simulink model "Sim7"  (R2021b)
settings: Solver=FixedStepDiscrete  StartTime=0.0  StopTime=1  FixedStep=1e-6  RelTol=1e-3  EnableMultiTasking=on
InitFcn:
  | clc
  | Ts=1e-6;
  | ts=Ts;
  | Td=Ts;
  | disp(sprintf('Ts = %f',Ts))
  |  %1/fs = sampling period;
  | Ts = Td;
  | Tch = Td;
  | 
  | %harmonics
  | kh=0;
  | 
  | % PLL
  | Tset = 0.1; % settling time
  | zeta = 0.707;   % damping ratio (optimized for best response of the second order TF
  | 
  | %grid params
  | tha = 0;
  | kh = 0;
  | V1 = 230;
  | fg = 50;
  | 
  | %freq var
  | onoff = 0;
  | onoff_faults = 1;
  | fperiod = 2;
  | fmin = 48;
  | fmax = 52;
undefined symbols (not defined in the file or in its folder): DiscIntNeverNeededParam
libraries: spsThreePhaseSeriesRLCBranchLib x8, powerlib_extras x5, spsThreePhaseVIMeasurementLib x5, spsSeriesRLCBranchLib x3, spsUniversalBridgeLib x3, spsGroundLib x2, spsDCVoltageSourceLib x2, spsThreePhaseBreakerLib x2, spspowerguiLib x1
(part 1 of 2)
settings Model: SimulationMode=accelerator  Creator=juancho  LastModifiedBy=sebastian
settings SolverCC: AlgebraicLoopSolver=TrustRegion
settings DataIOCC: SaveFormat=Array  SignalLoggingSaveFormat=ModelDataLogs  SaveOutput=off  SignalLogging=off  SaveTime=off  ReturnWorkspaceOutputs=off
settings OptimizationCC: ExpressionDepthLimit=2147483647  LifeSpan=inf
settings DebuggingCC: UnderspecifiedInitializationDetection=Classic  MergeDetectMultiDrivingBlocksExec=none  SolverPrmCheckMsg=warning  InheritedTsInSrcMsg=error  FcnCallInpInsideContextMsg=warning  AllowSymbolicDim=off  StateNameClashWarn=warning  SFUnexpectedBacktrackingDiag=warning  SFNoUnconditionalDefaultTransitionDiag=warning  SFExecutionAtInitializationDiag=none  SFMachineParentedDataDiag=warning  ArithmeticOperatorsInVariantConditions=warning
settings HardwareCC: ProdBitPerPointer=32  ProdBitPerSizeT=32  ProdBitPerPtrDiffT=32  ProdLargestAtomicFloat=None  ProdIntDivRoundTo=Undefined  ProdEndianess=Unspecified  ProdWordSize=32  ProdHWDeviceType=32-bit Generic
settings ModelReferenceCC: PropagateSignalLabelsOutOfModel=off
settings SFSimCC: SimUseLocalCustomCode=off  CustomCodeUndefinedFunction=UseInterfaceOnly
settings RTWCC: RTWUseLocalCustomCode=off
settings CodeAppCC: StateflowObjectComments=on
settings GRTTargetCC: TargetLangStandard=C89/C90 (ANSI)  CombineOutputUpdateFcns=off  GRTInterface=on
settings ConfigComp: CovMetricSettings=dw  CovSaveCumulativeToWorkspaceVar=on  CovSaveSingleToWorkspaceVar=on  CovExternalEMLEnable=off  CovSFcnEnable=off
settings SimscapeCC: SimscapeNormalizeSystem=off

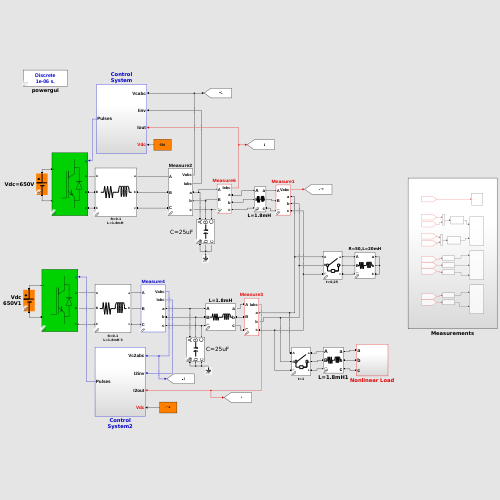
[thumbnail: Simulink's stored preview of the top-level diagram]
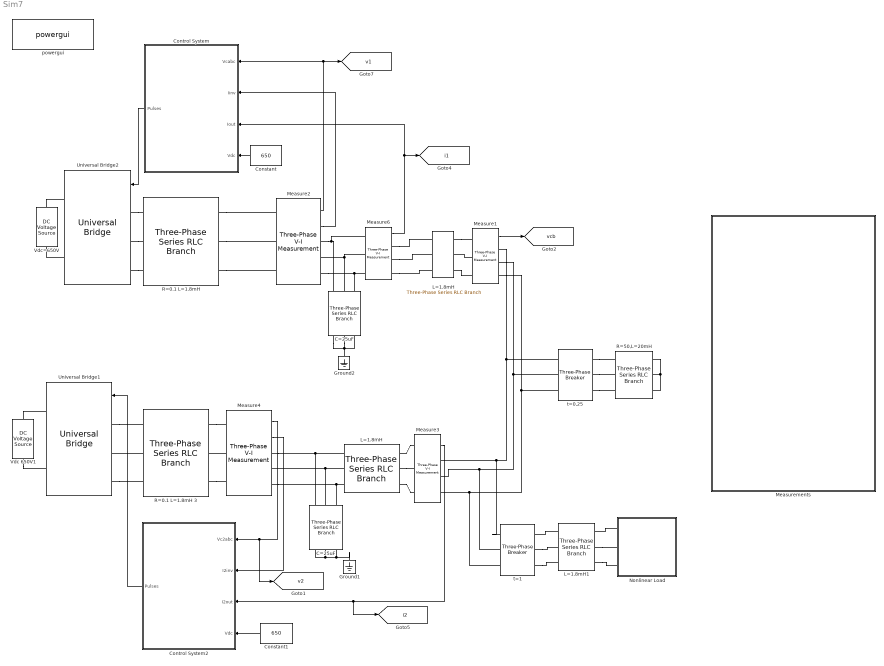
== system Sim7 ==
  C=25uF : spsThreePhaseSeriesRLCBranchLib/Three-Phase Series RLC Branch  LConnTagsString=A|B|C  RConnTagsString=A|B|C  BranchType=C  Resistance=1.0  Inductance=1e-3  Capacitance=25e-6  Measurements=None
  "C=25uF " : spsThreePhaseSeriesRLCBranchLib/Three-Phase Series RLC Branch  LConnTagsString=A|B|C  RConnTagsString=A|B|C  BranchType=C  Resistance=1.0  Inductance=1e-3  Capacitance=25e-6  Measurements=None
  Constant : Constant  Value=650
  Constant1 : Constant  Value=650
  Control System : Subsystem
  Control System2 : Subsystem
  Ground1 : spsGroundLib/Ground  LConnTagsString=a
  Ground2 : spsGroundLib/Ground  LConnTagsString=a
  L=1.8mH : spsThreePhaseSeriesRLCBranchLib/Three-Phase Series RLC Branch  LConnTagsString=A|B|C  RConnTagsString=A|B|C  BranchType=RL  Resistance=0.1  Inductance=1.8e-3  Capacitance=1.0  Measurements=None
  "L=1.8mH " : spsThreePhaseSeriesRLCBranchLib/Three-Phase Series RLC Branch  LConnTagsString=A|B|C  RConnTagsString=A|B|C  BranchType=RL  Resistance=0.1  Inductance=1.8e-3  Capacitance=1.0  Measurements=None
  L=1.8mH1 : spsThreePhaseSeriesRLCBranchLib/Three-Phase Series RLC Branch  LConnTagsString=A|B|C  RConnTagsString=A|B|C  BranchType=RL  Resistance=0.1  Inductance=(1.8e-3)  Capacitance=1.0  Measurements=None
  Measure1 : spsThreePhaseVIMeasurementLib/Three-Phase V-I Measurement  VoltageMeasurement=phase-to-ground  SetLabelV=off  LabelV=V1  Vpu=off  VpuLL=off  CurrentMeasurement=no  SetLabelI=off  LabelI=I1  Ipu=off  Pbase=1e3  Vbase=380  OutputType=Magnitude  PhasorSimulation=off  PSBequivalent=0
  Measure2 : spsThreePhaseVIMeasurementLib/Three-Phase V-I Measurement  VoltageMeasurement=phase-to-ground  SetLabelV=off  LabelV=V1  Vpu=off  VpuLL=off  CurrentMeasurement=yes  SetLabelI=off  LabelI=I1  Ipu=off  Pbase=1e3  Vbase=380  OutputType=Magnitude  PhasorSimulation=off  PSBequivalent=0
  Measure3 : spsThreePhaseVIMeasurementLib/Three-Phase V-I Measurement  VoltageMeasurement=no  SetLabelV=off  LabelV=V1  Vpu=off  VpuLL=off  CurrentMeasurement=yes  SetLabelI=off  LabelI=I1  Ipu=off  Pbase=1e3  Vbase=380  OutputType=Magnitude  PhasorSimulation=off  PSBequivalent=0
  Measure4 : spsThreePhaseVIMeasurementLib/Three-Phase V-I Measurement  VoltageMeasurement=phase-to-ground  SetLabelV=off  LabelV=V1  Vpu=off  VpuLL=off  CurrentMeasurement=yes  SetLabelI=off  LabelI=I1  Ipu=off  Pbase=1e3  Vbase=380  OutputType=Magnitude  PhasorSimulation=off  PSBequivalent=0
  Measure6 : spsThreePhaseVIMeasurementLib/Three-Phase V-I Measurement  VoltageMeasurement=no  SetLabelV=off  LabelV=V1  Vpu=off  VpuLL=off  CurrentMeasurement=yes  SetLabelI=off  LabelI=I1  Ipu=off  Pbase=1e3  Vbase=380  OutputType=Magnitude  PhasorSimulation=off  PSBequivalent=0
  Measurements : Subsystem
  Nonlinear Load : Subsystem
  "R=0.1 L=1.8mH " : spsThreePhaseSeriesRLCBranchLib/Three-Phase Series RLC Branch  LConnTagsString=A|B|C  RConnTagsString=A|B|C  BranchType=RL  Resistance=0.1  Inductance=1.8e-3  Capacitance=1.0  Measurements=None
  R=0.1 L=1.8mH 3 : spsThreePhaseSeriesRLCBranchLib/Three-Phase Series RLC Branch  LConnTagsString=A|B|C  RConnTagsString=A|B|C  BranchType=RL  Resistance=0.1  Inductance=1.8e-3  Capacitance=1.0  Measurements=None
  R=50,L=20mH : spsThreePhaseSeriesRLCBranchLib/Three-Phase Series RLC Branch  LConnTagsString=A|B|C  RConnTagsString=A|B|C  BranchType=RL  Resistance=50  Inductance=20e-3  Capacitance=1.0  Measurements=None
  Universal Bridge1 : spsUniversalBridgeLib/Universal Bridge  Arms=3  SnubberResistance=1e5  SnubberCapacitance=inf  Device=IGBT / Diodes  Ron=1e-3  Lon=0  ForwardVoltages="[  0  0  ]"  ForwardVoltage=0  GTOparameters=[ 10e-6 , 20e-6 ]  IGBTparameters=[ 1e-6 , 2e-6]  Measurements=None  Measurements_2=None  converterType=Rectifier
  Universal Bridge2 : spsUniversalBridgeLib/Universal Bridge  Arms=3  SnubberResistance=1e5  SnubberCapacitance=inf  Device=IGBT / Diodes  Ron=1e-3  Lon=0  ForwardVoltages="[  0  0  ]"  ForwardVoltage=0  GTOparameters=[ 10e-6 , 20e-6 ]  IGBTparameters=[ 1e-6 , 2e-6 ]  Measurements=None  Measurements_2=None  converterType=Rectifier
  Vdc 650V1 : spsDCVoltageSourceLib/DC Voltage Source  Description=source block  Amplitude=650  Measurements=None
      settings: AttributesFormatString=\n
  Vdc=650V : spsDCVoltageSourceLib/DC Voltage Source  Description=source block  Amplitude=650  Measurements=None
      settings: AttributesFormatString=\n
  powergui : spspowerguiLib/powergui  Priority=1  SimulationMode=Discrete  SampleTime=1e-6  frequency=60  Iterations=50  frequencyindice=0  Pbase=100e6  ErrMax=1e-4  UnitsV=kV  UnitsW=MW  buscounter=0  FunctionMessages=off  echomessages=off  EnableUseOfTLC=off  CurrentSourceSwitches=off  DisableSnubberDevices=off  DisableRonSwitches=off  DisableVfSwitches=off  DisplayEquations=off  AutomaticDiscreteSolvers=off  SolverType=Tustin  Interpol=off  ExternalGateDelay=off  methode=off  Ts=0  x0status=blocks  SPID=off  SwTol=0  HookPort=off  NonlinearTolerance=1e-4  nMaxIteration=100  ContinueOnMaxIteration=off  RestoreLinks=warning  ResistiveCurrentMeasurement=off  Frange=[0:2:500]  Ylog=off  Xlog=on  ShowGrid=off  save=off  variable=ZData  structure=vload  ZoomFFT=off  StartTime=4.8  cycles=9  DisplayStyle=1  fundamental=49.953  FreqAxis=on  MaxFrequency=1000  frequencyindicesteady=1  RmsSteady=1  display=off
  "t=0,25 " : spsThreePhaseBreakerLib/Three-Phase Breaker  InitialState=open  SwitchA=on  SwitchB=on  SwitchC=on  SwitchTimes=0.25  External=off  BreakerResistance=0.001  SnubberResistance=1e6  SnubberCapacitance=inf  Measurements=None
  t=1 : spsThreePhaseBreakerLib/Three-Phase Breaker  InitialState=open  SwitchA=on  SwitchB=on  SwitchC=on  SwitchTimes=1  External=off  BreakerResistance=0.001  SnubberResistance=1e6  SnubberCapacitance=inf  Measurements=Breaker voltages and currents
  tag scope: i1=global, i2=global, v1=global, v2=global, vcb=global
  wires:
  Control System/1(Pulses) -> Universal Bridge2/1
  Constant/1 -> Control System/4(Vdc)
  Measure2/1 -> Control System/1(Vcabc), [v1]
  Measure4/1 -> [v2], Control System2/1(Vc2abc)
  Control System2/1(Pulses) -> Universal Bridge1/1
  Measure4/2 -> Control System2/2(I2inv)
  Measure3/1 -> [i2], Control System2/3(I2out)
  Constant1/1 -> Control System2/4(Vdc)
  Measure2/2 -> Control System/2(Iinv)
  Measure6/1 -> [i1], Control System/3(Iout)
  Measure1/1 -> [vcb]
  connections:
  Universal Bridge2/LConn3 -- "R=0.1 L=1.8mH "/LConn3
  Universal Bridge2/LConn1 -- "R=0.1 L=1.8mH "/LConn1
  Universal Bridge2/LConn2 -- "R=0.1 L=1.8mH "/LConn2
  Universal Bridge2/RConn2 -- Vdc=650V/LConn1
  Vdc=650V/RConn1 -- Universal Bridge2/RConn1
  "R=0.1 L=1.8mH "/RConn1 -- Measure2/LConn1
  "R=0.1 L=1.8mH "/RConn2 -- Measure2/LConn2
  "R=0.1 L=1.8mH "/RConn3 -- Measure2/LConn3
  "C=25uF "/RConn2 -- Ground2/LConn1 -- "C=25uF "/RConn1 -- "C=25uF "/RConn3
  Measure1/RConn2 -- t=1/LConn2 -- Measure3/RConn2 -- "t=0,25 "/LConn2
  Measure1/RConn3 -- t=1/LConn3 -- Measure3/RConn3 -- "t=0,25 "/LConn3
  Universal Bridge1/LConn1 -- R=0.1 L=1.8mH 3/LConn1
  R=0.1 L=1.8mH 3/LConn2 -- Universal Bridge1/LConn2
  Universal Bridge1/LConn3 -- R=0.1 L=1.8mH 3/LConn3
  R=0.1 L=1.8mH 3/RConn1 -- Measure4/LConn1
  Measure4/LConn2 -- R=0.1 L=1.8mH 3/RConn2
  R=0.1 L=1.8mH 3/RConn3 -- Measure4/LConn3
  Measure4/RConn1 -- L=1.8mH/LConn1 -- C=25uF/LConn1
  L=1.8mH/LConn2 -- Measure4/RConn2 -- C=25uF/LConn2
  L=1.8mH/RConn1 -- Measure3/LConn1
  L=1.8mH/RConn2 -- Measure3/LConn2
  L=1.8mH/RConn3 -- Measure3/LConn3
  Measure1/RConn1 -- "t=0,25 "/LConn1 -- t=1/LConn1 -- Measure3/RConn1
  Measure2/RConn3 -- Measure6/LConn3 -- "C=25uF "/LConn3
  Measure2/RConn1 -- Measure6/LConn1 -- "C=25uF "/LConn1
  "C=25uF "/LConn2 -- Measure6/LConn2 -- Measure2/RConn2
  C=25uF/RConn3 -- C=25uF/RConn1 -- C=25uF/RConn2 -- Ground1/LConn1
  Measure4/RConn3 -- L=1.8mH/LConn3 -- C=25uF/LConn3
  Vdc 650V1/LConn1 -- Universal Bridge1/RConn2
  Vdc 650V1/RConn1 -- Universal Bridge1/RConn1
  R=50,L=20mH/RConn2 -- R=50,L=20mH/RConn1 -- R=50,L=20mH/RConn3
  "t=0,25 "/RConn1 -- R=50,L=20mH/LConn1
  "t=0,25 "/RConn2 -- R=50,L=20mH/LConn2
  "L=1.8mH "/RConn1 -- Measure1/LConn1
  Measure1/LConn2 -- "L=1.8mH "/RConn2
  "L=1.8mH "/RConn3 -- Measure1/LConn3
  Measure6/RConn1 -- "L=1.8mH "/LConn1
  Measure6/RConn2 -- "L=1.8mH "/LConn2
  Measure6/RConn3 -- "L=1.8mH "/LConn3
  "t=0,25 "/RConn3 -- R=50,L=20mH/LConn3
  L=1.8mH1/RConn2 -- Nonlinear Load/LConn2
  L=1.8mH1/LConn1 -- t=1/RConn1
  t=1/RConn2 -- L=1.8mH1/LConn2
  Nonlinear Load/LConn1 -- L=1.8mH1/RConn1
  L=1.8mH1/RConn3 -- Nonlinear Load/LConn3
  t=1/RConn3 -- L=1.8mH1/LConn3

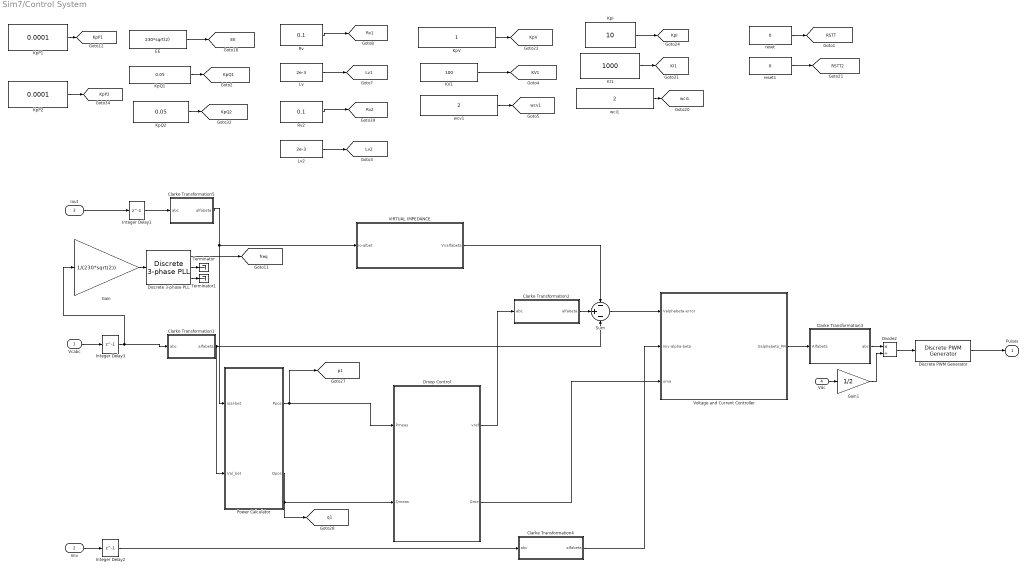
== system Sim7/Control System ==
  Vcabc : Inport
  Iinv : Inport  Port=2
  Iout : Inport  Port=3
  Vdc : Inport  Port=4
  Clarke Transformation3 : Subsystem
  Clarke Transformation1 : Subsystem
  Clarke Transformation2 : Subsystem
  Clarke Transformation4 : Subsystem
  Clarke Transformation5 : Subsystem
  Discrete 3-phase PLL : powerlib_extras/Discrete  Control Blocks/Discrete 3-phase PLL  Fmin=45  Par_Init=[0 50]  ParK=[ 180 3200 1 ]  Ts=1e-6  AGC=off
      settings: SourceProductBaseCode=PS
  Discrete PWM Generator : powerlib_extras/Discrete  Control Blocks/Discrete PWM Generator  GeneratorMode="3-arm  bridge (6 pulses)"  Fc=1e4  Ts=1e-6  Internal=off  mIndex=0.4  Freq=60  Phase=0
      settings: SourceProductBaseCode=PS
  Divide2 : Product  Inputs=*/  SampleTime=Ts
  Droop Control : Subsystem
  EE : Constant  Value=230*sqrt(2)
  Gain : Gain  Gain=1/(230*sqrt(2))
  Gain1 : Gain  Gain=1/2  SampleTime=Ts
  Integer Delay1 : Delay  DelayLength=1  SampleTime=1e-6
  Integer Delay2 : Delay  DelayLength=1  SampleTime=1e-6
  Integer Delay3 : Delay  DelayLength=1  SampleTime=1e-6
  KI1 : Constant  Value=1000
  KV1 : Constant  Value=100
  KpI : Constant  Value=10
  KpP1 : Constant  Value=0.0001
  KpP2 : Constant  Value=0.0001
  KpQ1 : Constant  Value=0.05  VectorParams1D=off
  KpQ2 : Constant  Value=0.05  VectorParams1D=off
  KpV : Constant
  Lv : Constant  Value=2e-3
  Lv2 : Constant  Value=2e-3
  Power Calculator : Subsystem
  Rv : Constant  Value=0.1
  Rv2 : Constant  Value=0.1
  Sum : Sum  Inputs=-+-  SampleTime=Ts
  Terminator : Terminator
  Terminator1 : Terminator
  VIRTUAL IMPEDANCE : Subsystem
  "Voltage and Current Controller " : Subsystem
  reset : Constant  Value=0
  reset1 : Constant  Value=0
  wci1 : Constant  Value=2
  wcv1 : Constant  Value=2
  Pulses : Outport  SampleTime=1e-6
  tag scope: EE=global, KI1=global, KV1=global, KpI=global, KpP1=global, KpP2=global, KpQ1=global, KpQ2=global, KpV=global, Lv1=global, Lv2=global, RSTT2=global, RSTT=global, Rv1=global, Rv2=global, freq=global, p1=global, q1=global, wci1=global, wcv1=global
  wires:
  Lv/1 -> [Lv1]
  Rv/1 -> [Rv1]
  KpP1/1 -> [KpP1]
  KpQ1/1 -> [KpQ1]
  EE/1 -> [EE]
  reset/1 -> [RSTT]
  Iinv/1 -> Integer Delay2/1
  Iout/1 -> Integer Delay1/1
  Vcabc/1 -> Integer Delay3/1
  Vdc/1 -> Gain1/1
  VIRTUAL IMPEDANCE/1(Vvalfabeta) -> Sum/1
  Clarke Transformation2/1(alfabeta) -> Sum/2
  Clarke Transformation5/1(alfabeta) -> Power Calculator/1(ioal-bet), VIRTUAL IMPEDANCE/1(io-albet)
  Clarke Transformation1/1(alfabeta) -> Sum/3, Power Calculator/2(Val_bet)
  Droop Control/2(Ome) -> "Voltage and Current Controller "/3(ome)
  Divide2/1 -> Discrete PWM Generator/1
  Gain1/1 -> Divide2/2
  Clarke Transformation3/1(abc) -> Divide2/1
  Discrete PWM Generator/1 -> Pulses/1
  Integer Delay2/1 -> Clarke Transformation4/1(abc)
  Integer Delay3/1 -> Clarke Transformation1/1(abc), Gain/1
  Integer Delay1/1 -> Clarke Transformation5/1(abc)
  Droop Control/1(vref) -> Clarke Transformation2/1(abc)
  Power Calculator/1(Ppos) -> [p1], Droop Control/1(Pmeas)
  Power Calculator/2(Qpos) -> Droop Control/2(Qmeas), [q1]
  reset1/1 -> [RSTT2]
  "Voltage and Current Controller "/1(Ualphabeta_PR) -> Clarke Transformation3/1(Alfabeta)
  Clarke Transformation4/1(alfabeta) -> "Voltage and Current Controller "/2(Iinv-alpha-beta)
  Sum/1 -> "Voltage and Current Controller "/1(Valphabeta-error)
  KpV/1 -> [KpV]
  KpI/1 -> [KpI]
  KI1/1 -> [KI1]
  KV1/1 -> [KV1]
  wcv1/1 -> [wcv1]
  wci1/1 -> [wci1]
  Gain/1 -> Discrete 3-phase PLL/1
  Discrete 3-phase PLL/1 -> [freq]
  KpQ2/1 -> [KpQ2]
  KpP2/1 -> [KpP2]
  Lv2/1 -> [Lv2]
  Rv2/1 -> [Rv2]
  Discrete 3-phase PLL/2 -> Terminator/1
  Discrete 3-phase PLL/3 -> Terminator1/1

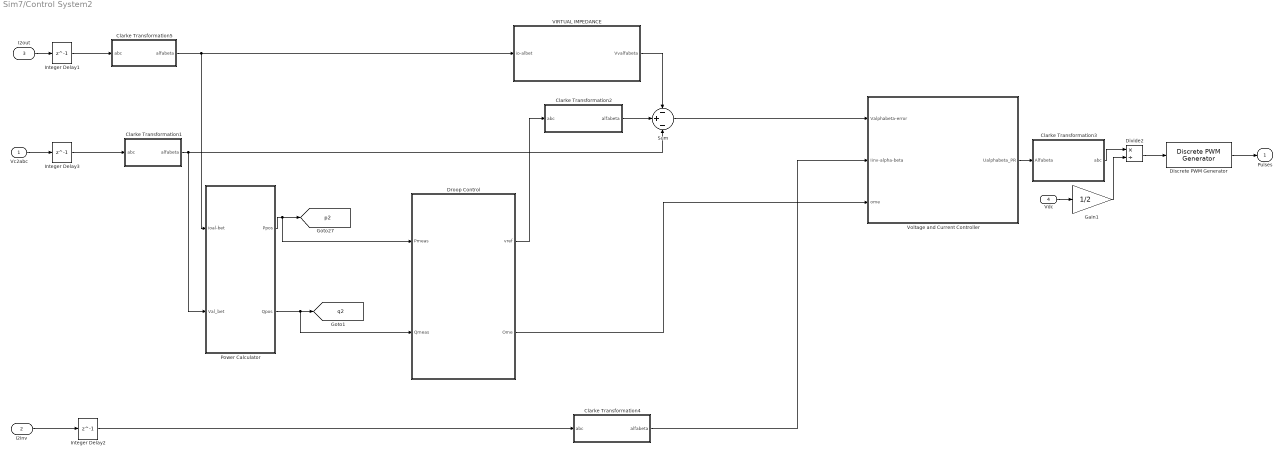
== system Sim7/Control System2 ==
  Vc2abc : Inport
  I2inv : Inport  Port=2
  I2out : Inport  Port=3
  Vdc : Inport  Port=4
  Clarke Transformation3 : Subsystem
  Clarke Transformation1 : Subsystem
  Clarke Transformation2 : Subsystem
  Clarke Transformation4 : Subsystem
  Clarke Transformation5 : Subsystem
  Discrete PWM Generator : powerlib_extras/Discrete  Control Blocks/Discrete PWM Generator  GeneratorMode="3-arm  bridge (6 pulses)"  Fc=1e4  Ts=1e-6  Internal=off  mIndex=0.4  Freq=60  Phase=0
      settings: SourceProductBaseCode=PS
  Divide2 : Product  Inputs=*/  SampleTime=Ts
  Droop Control : Subsystem
  Gain1 : Gain  Gain=1/2  SampleTime=Ts
  Integer Delay1 : Delay  DelayLength=1  SampleTime=1e-6
  Integer Delay2 : Delay  DelayLength=1  SampleTime=1e-6
  Integer Delay3 : Delay  DelayLength=1  SampleTime=1e-6
  Power Calculator : Subsystem
  Sum : Sum  Inputs=-+-  SampleTime=Ts
  VIRTUAL IMPEDANCE : Subsystem
  Voltage and Current Controller : Subsystem
  Pulses : Outport  SampleTime=1e-6
  tag scope: p2=global, q2=global
  wires:
  Droop Control/2(Ome) -> Voltage and Current Controller/3(ome)
  Clarke Transformation1/1(alfabeta) -> Sum/3, Power Calculator/2(Val_bet)
  Clarke Transformation3/1(abc) -> Divide2/1
  Clarke Transformation2/1(alfabeta) -> Sum/2
  VIRTUAL IMPEDANCE/1(Vvalfabeta) -> Sum/1
  Gain1/1 -> Divide2/2
  Vc2abc/1 -> Integer Delay3/1
  I2out/1 -> Integer Delay1/1
  Integer Delay2/1 -> Clarke Transformation4/1(abc)
  I2inv/1 -> Integer Delay2/1
  Vdc/1 -> Gain1/1
  Divide2/1 -> Discrete PWM Generator/1
  Discrete PWM Generator/1 -> Pulses/1
  Integer Delay3/1 -> Clarke Transformation1/1(abc)
  Integer Delay1/1 -> Clarke Transformation5/1(abc)
  Clarke Transformation5/1(alfabeta) -> VIRTUAL IMPEDANCE/1(io-albet), Power Calculator/1(ioal-bet)
  Power Calculator/1(Ppos) -> Droop Control/1(Pmeas), [p2]
  Power Calculator/2(Qpos) -> Droop Control/2(Qmeas), [q2]
  Droop Control/1(vref) -> Clarke Transformation2/1(abc)
  Voltage and Current Controller/1(Ualphabeta_PR) -> Clarke Transformation3/1(Alfabeta)
  Clarke Transformation4/1(alfabeta) -> Voltage and Current Controller/2(Iinv-alpha-beta)
  Sum/1 -> Voltage and Current Controller/1(Valphabeta-error)

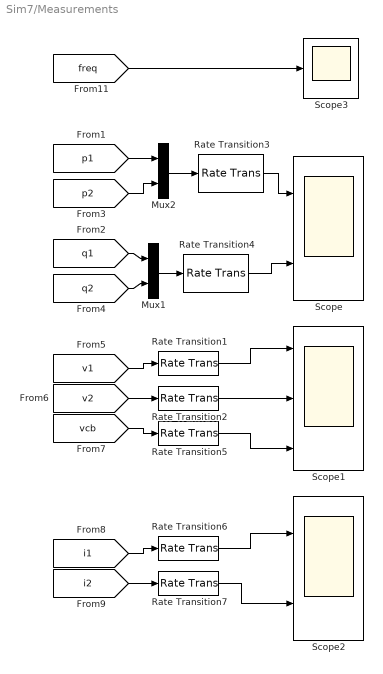
== system Sim7/Measurements ==
  Mux1 : Mux  Inputs=2
  Mux2 : Mux  Inputs=2
  Rate Transition{1..7} (7 alike) : RateTransition  OutPortSampleTime=1e-4
  Scope : Scope  NumInputPorts=2
  Scope1 : Scope  NumInputPorts=3
  Scope2 : Scope  NumInputPorts=2
  Scope3 : Scope
  wires:
  [p2] -> Mux2/2
  Rate Transition2/1 -> Scope1/2
  Rate Transition7/1 -> Scope2/2
  [v1] -> Rate Transition1/1
  Rate Transition1/1 -> Scope1/1
  [v2] -> Rate Transition2/1
  Rate Transition5/1 -> Scope1/3
  [q1] -> Mux1/1
  [p1] -> Mux2/1
  [i1] -> Rate Transition6/1
  Rate Transition3/1 -> Scope/1
  Mux1/1 -> Rate Transition4/1
  [q2] -> Mux1/2
  Mux2/1 -> Rate Transition3/1
  Rate Transition4/1 -> Scope/2
  Rate Transition6/1 -> Scope2/1
  [i2] -> Rate Transition7/1
  [vcb] -> Rate Transition5/1
  [freq] -> Scope3/1

== system Sim7/Nonlinear Load ==
  84uH : spsSeriesRLCBranchLib/Series RLC Branch  LConnTagsString=__new0  RConnTagsString=__new0  BranchType=L  Resistance=1  Inductance=84e-6  SetiL0=off  InitialCurrent=0  Capacitance=1e-6  Setx0=off  InitialVoltage=0  Measurements=None
  C 235uF : spsSeriesRLCBranchLib/Series RLC Branch  LConnTagsString=__new0  RConnTagsString=__new0  BranchType=C  Resistance=10e3  Inductance=[]  SetiL0=off  InitialCurrent=0  Capacitance=235e-6  Setx0=off  InitialVoltage=0  Measurements=None
  R 50 Ohms : spsSeriesRLCBranchLib/Series RLC Branch  LConnTagsString=__new0  RConnTagsString=__new0  BranchType=R  Resistance=50  Inductance=1.8e-3  SetiL0=off  InitialCurrent=0  Capacitance=[]  Setx0=off  InitialVoltage=0  Measurements=None
  Universal Bridge : spsUniversalBridgeLib/Universal Bridge  Arms=3  SnubberResistance=1e5  SnubberCapacitance=1e-6  Device=Diodes  Ron=1e-3  Lon=0  ForwardVoltages="[  0  0  ]"  ForwardVoltage=0.8  GTOparameters=[ 10e-6 , 20e-6 ]  IGBTparameters=[ 1e-6 , 2e-6 ]  Measurements=All voltages and currents  Measurements_2=None  converterType=Rectifier
  a : PMIOPort  Side=Left
  b : PMIOPort  Port=2  Side=Left
  c : PMIOPort  Port=3  Side=Left
  connections:
  C 235uF/LConn1 -- R 50 Ohms/RConn1 -- Universal Bridge/RConn2
  R 50 Ohms/LConn1 -- 84uH/LConn1 -- C 235uF/RConn1
  Universal Bridge/LConn1 -- a/RConn1
  Universal Bridge/LConn3 -- c/RConn1
  Universal Bridge/LConn2 -- b/RConn1
  84uH/RConn1 -- Universal Bridge/RConn1

== system Sim7/Control System/Clarke Transformation3 ==
  Alfabeta : Inport  SampleTime=Ts
  A : Fcn  Expr=sqrt(2/3)*u[1]  SampleTime=Ts
  B : Fcn  Expr=sqrt(2/3)*((-1/2)*u[1] + (sqrt(3)/2)*u[2])  SampleTime=Ts
  C : Fcn  Expr=sqrt(2/3)*((-1/2)*u[1] - (sqrt(3)/2)*u[2])  SampleTime=Ts
  Mux1 : Mux  Inputs=3
  abc : Outport  SampleTime=Ts
  wires:
  C/1 -> Mux1/3
  Alfabeta/1 -> C/1, B/1, A/1
  B/1 -> Mux1/2
  A/1 -> Mux1/1
  Mux1/1 -> abc/1

== system Sim7/Control System/Clarke Transformation1 ==
  abc : Inport  SampleTime=Ts
  Clarke to Beta : Fcn  Expr=sqrt(2/3)*(0*u[1]+(sqrt(3)/2)*u[2]-(sqrt(3)/2)*u[3])  SampleTime=Ts
  Clarke to alpha : Fcn  Expr=sqrt(2/3)*(u[1]-(1/2)*u[2]-(1/2)*u[3])  SampleTime=Ts
  Mux1 : Mux  Inputs=2
  alfabeta : Outport  SampleTime=Ts
  wires:
  abc/1 -> Clarke to Beta/1, Clarke to alpha/1
  Mux1/1 -> alfabeta/1
  Clarke to alpha/1 -> Mux1/1
  Clarke to Beta/1 -> Mux1/2

== system Sim7/Control System/Clarke Transformation2 ==
  abc : Inport  SampleTime=Ts
  Clarke to Beta : Fcn  Expr=sqrt(2/3)*(0*u[1]+(sqrt(3)/2)*u[2]-(sqrt(3)/2)*u[3])  SampleTime=Ts
  Clarke to alpha : Fcn  Expr=sqrt(2/3)*(u[1]-(1/2)*u[2]-(1/2)*u[3])  SampleTime=Ts
  Mux1 : Mux  Inputs=2
  alfabeta : Outport  SampleTime=Ts
  wires:
  Clarke to Beta/1 -> Mux1/2
  Clarke to alpha/1 -> Mux1/1
  Mux1/1 -> alfabeta/1
  abc/1 -> Clarke to alpha/1, Clarke to Beta/1

== system Sim7/Control System/Clarke Transformation4 ==
  abc : Inport  SampleTime=Ts
  Clarke to Beta : Fcn  Expr=sqrt(2/3)*(0*u[1]+(sqrt(3)/2)*u[2]-(sqrt(3)/2)*u[3])  SampleTime=Ts
  Clarke to alpha : Fcn  Expr=sqrt(2/3)*(u[1]-(1/2)*u[2]-(1/2)*u[3])  SampleTime=Ts
  Mux1 : Mux  Inputs=2
  alfabeta : Outport  SampleTime=Ts
  wires:
  Clarke to Beta/1 -> Mux1/2
  Clarke to alpha/1 -> Mux1/1
  Mux1/1 -> alfabeta/1
  abc/1 -> Clarke to alpha/1, Clarke to Beta/1

== system Sim7/Control System/Clarke Transformation5 ==
  abc : Inport  SampleTime=Ts
  Clarke to Beta : Fcn  Expr=sqrt(2/3)*(0*u[1]+(sqrt(3)/2)*u[2]-(sqrt(3)/2)*u[3])  SampleTime=Ts
  Clarke to alpha : Fcn  Expr=sqrt(2/3)*(u[1]-(1/2)*u[2]-(1/2)*u[3])  SampleTime=Ts
  Mux1 : Mux  Inputs=2
  alfabeta : Outport  SampleTime=Ts
  wires:
  abc/1 -> Clarke to Beta/1, Clarke to alpha/1
  Mux1/1 -> alfabeta/1
  Clarke to alpha/1 -> Mux1/1
  Clarke to Beta/1 -> Mux1/2

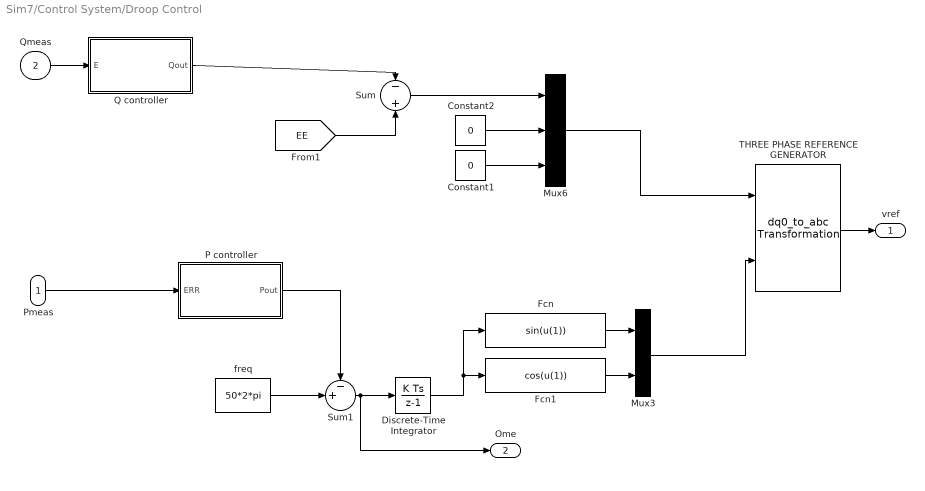
== system Sim7/Control System/Droop Control ==
  Pmeas : Inport  SampleTime=Ts
  Qmeas : Inport  Port=2  SampleTime=Ts
  Constant1 : Constant  Value=0
  Constant2 : Constant  Value=0
  Discrete-Time Integrator : DiscreteIntegrator  SampleTime=-1  ICPrevOutput=DiscIntNeverNeededParam  ICPrevScaledInput=DiscIntNeverNeededParam
  Fcn : Fcn  Expr=sin(u(1))
  Fcn1 : Fcn  Expr=cos(u(1))
  Mux3 : Mux  Inputs=2
  Mux6 : Mux  Inputs=3
  P controller : Subsystem
  Q controller : Subsystem
  Sum : Sum  Inputs=-|+  SampleTime=Ts
  Sum1 : Sum  Inputs=-+|
  THREE PHASE REFERENCE GENERATOR : powerlib_extras/Measurements/dq0_to_abc Transformation
      settings: SourceProductBaseCode=PS
  freq : Constant  Value=50*2*pi
  vref : Outport  SampleTime=Ts
  Ome : Outport  Port=2  SampleTime=Ts
  wires:
  Pmeas/1 -> P controller/1(ERR)
  Qmeas/1 -> Q controller/1(E)
  Constant2/1 -> Mux6/2
  Constant1/1 -> Mux6/3
  Mux6/1 -> THREE PHASE REFERENCE GENERATOR/1
  Fcn/1 -> Mux3/1
  Fcn1/1 -> Mux3/2
  THREE PHASE REFERENCE GENERATOR/1 -> vref/1
  Mux3/1 -> THREE PHASE REFERENCE GENERATOR/2
  Q controller/1(Qout) -> Sum/1
  P controller/1(Pout) -> Sum1/1
  [EE] -> Sum/2
  Sum/1 -> Mux6/1
  Sum1/1 -> Ome/1, Discrete-Time Integrator/1
  freq/1 -> Sum1/2
  Discrete-Time Integrator/1 -> Fcn/1, Fcn1/1

== system Sim7/Control System/Power Calculator ==
  ioal-bet : Inport
  Val_bet : Inport  Port=2
  Filter 1Hz 1MHz : Subsystem  Tag=FilterWizardSubSystem
      settings: ErrorFcn=dspFilterRealizedInBasicElemsAlgLoopErrFcnCallback
  Filter 1Hz 1MHz1 : Subsystem  Tag=FilterWizardSubSystem
      settings: ErrorFcn=dspFilterRealizedInBasicElemsAlgLoopErrFcnCallback
  Instantaneous active power1 : Fcn  Expr=u(1)*u(3)+u(2)*u(4)
  Instantaneous reactive power1 : Fcn  Expr=(-u(1)*u(4)+u(2)*u(3))
  Mux9 : Mux  Inputs=2
  Ppos : Outport
  Qpos : Outport  Port=2
  wires:
  Instantaneous active power1/1 -> Filter 1Hz 1MHz/1(Input)
  Mux9/1 -> Instantaneous active power1/1, Instantaneous reactive power1/1
  Instantaneous reactive power1/1 -> Filter 1Hz 1MHz1/1(Input)
  Val_bet/1 -> Mux9/1
  ioal-bet/1 -> Mux9/2
  Filter 1Hz 1MHz/1(Output) -> Ppos/1
  Filter 1Hz 1MHz1/1(Output) -> Qpos/1

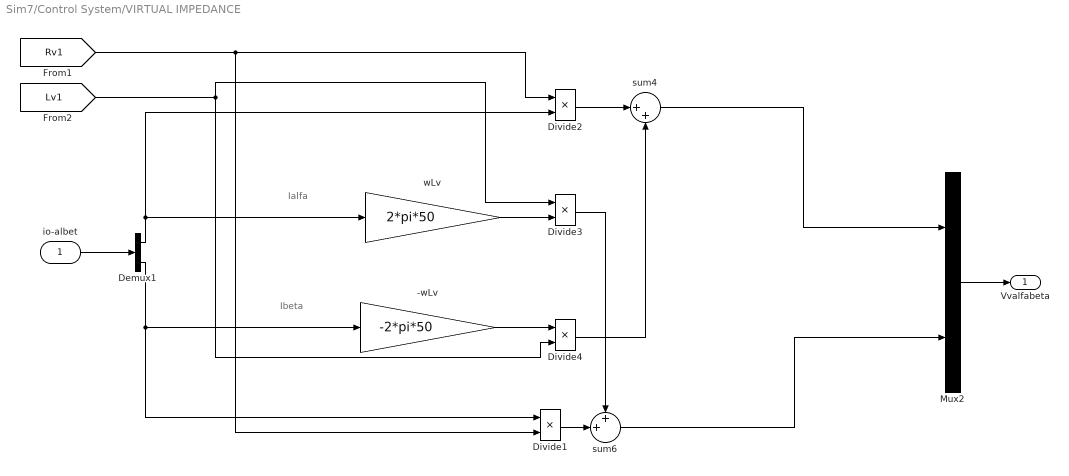
== system Sim7/Control System/VIRTUAL IMPEDANCE ==
  note: Ialfa
  note: Ibeta
  io-albet : Inport
  -wLv : Gain  Gain=-2*pi*50
  Demux1 : Demux  Outputs=2
  Divide{1..4} (4 alike) : Product  Inputs=**  OutDataTypeStr=Inherit: Same as first input
  Mux2 : Mux  Inputs=2
  sum4 : Sum  Inputs=|++  InputSameDT=on  SaturateOnIntegerOverflow=on  OutDataTypeStr=Inherit: Same as first input
  sum6 : Sum  Inputs=++|  InputSameDT=on  SaturateOnIntegerOverflow=on  OutDataTypeStr=Inherit: Same as first input
  wLv : Gain  Gain=2*pi*50
  Vvalfabeta : Outport
  wires:
  Divide2/1 -> sum4/1
  Divide1/1 -> sum6/2
  wLv/1 -> Divide3/2
  Divide3/1 -> sum6/1
  [Lv1] -> Divide3/1, Divide4/2
  -wLv/1 -> Divide4/1
  Divide4/1 -> sum4/2
  Mux2/1 -> Vvalfabeta/1
  Demux1/2 -> -wLv/1, Divide1/1
  Demux1/1 -> wLv/1, Divide2/2
  [Rv1] -> Divide2/1, Divide1/2
  sum6/1 -> Mux2/2
  io-albet/1 -> Demux1/1
  sum4/1 -> Mux2/1

== system Sim7/Control System/Voltage and Current Controller  ==
  Valphabeta-error : Inport
  Iinv-alpha-beta : Inport  Port=2
  ome : Inport  Port=3
  Current Controller : Subsystem
  Sum3 : Sum  Inputs=|+-  SaturateOnIntegerOverflow=on
  Voltage Controller : Subsystem
  Ualphabeta_PR : Outport
  wires:
  Iinv-alpha-beta/1 -> Sum3/2
  ome/1 -> Current Controller/2(Ome), Voltage Controller/2(Ome)
  Valphabeta-error/1 -> Voltage Controller/1(Val_bet-error)
  Current Controller/1(Valbet-ref) -> Ualphabeta_PR/1
  Sum3/1 -> Current Controller/1(Ial_bet-error)
  Voltage Controller/1(Ialbet-ref) -> Sum3/1

== system Sim7/Control System2/Clarke Transformation3 ==
  Alfabeta : Inport  SampleTime=Ts
  A : Fcn  Expr=sqrt(2/3)*u[1]  SampleTime=Ts
  B : Fcn  Expr=sqrt(2/3)*((-1/2)*u[1] + (sqrt(3)/2)*u[2])  SampleTime=Ts
  C : Fcn  Expr=sqrt(2/3)*((-1/2)*u[1] - (sqrt(3)/2)*u[2])  SampleTime=Ts
  Mux1 : Mux  Inputs=3
  abc : Outport  SampleTime=Ts
  wires:
  Mux1/1 -> abc/1
  A/1 -> Mux1/1
  B/1 -> Mux1/2
  Alfabeta/1 -> A/1, B/1, C/1
  C/1 -> Mux1/3

== system Sim7/Control System2/Clarke Transformation1 ==
  abc : Inport  SampleTime=Ts
  Clarke to Beta : Fcn  Expr=sqrt(2/3)*(0*u[1]+(sqrt(3)/2)*u[2]-(sqrt(3)/2)*u[3])  SampleTime=Ts
  Clarke to alpha : Fcn  Expr=sqrt(2/3)*(u[1]-(1/2)*u[2]-(1/2)*u[3])  SampleTime=Ts
  Mux1 : Mux  Inputs=2
  alfabeta : Outport  SampleTime=Ts
  wires:
  Clarke to Beta/1 -> Mux1/2
  Clarke to alpha/1 -> Mux1/1
  Mux1/1 -> alfabeta/1
  abc/1 -> Clarke to alpha/1, Clarke to Beta/1

== system Sim7/Control System2/Clarke Transformation2 ==
  abc : Inport  SampleTime=Ts
  Clarke to Beta : Fcn  Expr=sqrt(2/3)*(0*u[1]+(sqrt(3)/2)*u[2]-(sqrt(3)/2)*u[3])  SampleTime=Ts
  Clarke to alpha : Fcn  Expr=sqrt(2/3)*(u[1]-(1/2)*u[2]-(1/2)*u[3])  SampleTime=Ts
  Mux1 : Mux  Inputs=2
  alfabeta : Outport  SampleTime=Ts
  wires:
  abc/1 -> Clarke to Beta/1, Clarke to alpha/1
  Mux1/1 -> alfabeta/1
  Clarke to alpha/1 -> Mux1/1
  Clarke to Beta/1 -> Mux1/2

== system Sim7/Control System2/Clarke Transformation4 ==
  abc : Inport  SampleTime=Ts
  Clarke to Beta : Fcn  Expr=sqrt(2/3)*(0*u[1]+(sqrt(3)/2)*u[2]-(sqrt(3)/2)*u[3])  SampleTime=Ts
  Clarke to alpha : Fcn  Expr=sqrt(2/3)*(u[1]-(1/2)*u[2]-(1/2)*u[3])  SampleTime=Ts
  Mux1 : Mux  Inputs=2
  alfabeta : Outport  SampleTime=Ts
  wires:
  abc/1 -> Clarke to Beta/1, Clarke to alpha/1
  Mux1/1 -> alfabeta/1
  Clarke to alpha/1 -> Mux1/1
  Clarke to Beta/1 -> Mux1/2

== system Sim7/Control System2/Clarke Transformation5 ==
  abc : Inport  SampleTime=Ts
  Clarke to Beta : Fcn  Expr=sqrt(2/3)*(0*u[1]+(sqrt(3)/2)*u[2]-(sqrt(3)/2)*u[3])  SampleTime=Ts
  Clarke to alpha : Fcn  Expr=sqrt(2/3)*(u[1]-(1/2)*u[2]-(1/2)*u[3])  SampleTime=Ts
  Mux1 : Mux  Inputs=2
  alfabeta : Outport  SampleTime=Ts
  wires:
  Clarke to Beta/1 -> Mux1/2
  Clarke to alpha/1 -> Mux1/1
  Mux1/1 -> alfabeta/1
  abc/1 -> Clarke to alpha/1, Clarke to Beta/1

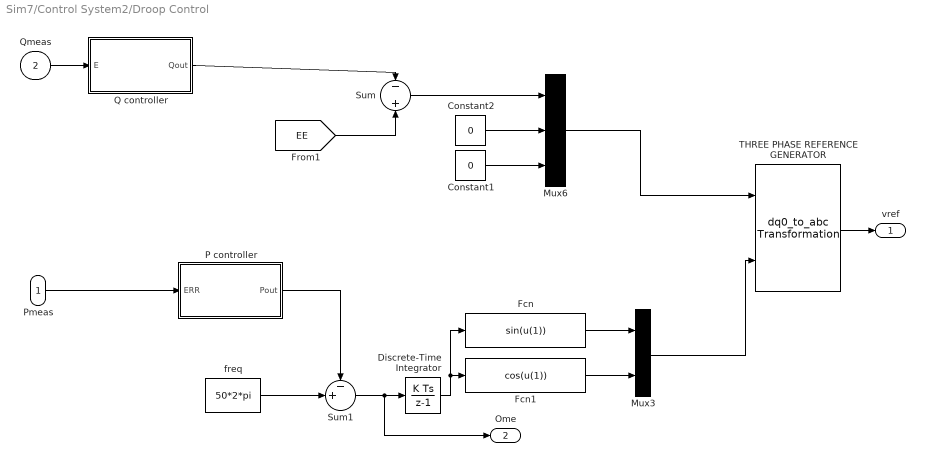
== system Sim7/Control System2/Droop Control ==
  Pmeas : Inport  SampleTime=Ts
  Qmeas : Inport  Port=2  SampleTime=Ts
  Constant1 : Constant  Value=0
  Constant2 : Constant  Value=0
  Discrete-Time Integrator : DiscreteIntegrator  SampleTime=-1  ICPrevOutput=DiscIntNeverNeededParam  ICPrevScaledInput=DiscIntNeverNeededParam
  Fcn : Fcn  Expr=sin(u(1))
  Fcn1 : Fcn  Expr=cos(u(1))
  Mux3 : Mux  Inputs=2
  Mux6 : Mux  Inputs=3
  P controller : Subsystem
  Q controller : Subsystem
  Sum : Sum  Inputs=-|+  SampleTime=Ts
  Sum1 : Sum  Inputs=-+|
  THREE PHASE REFERENCE GENERATOR : powerlib_extras/Measurements/dq0_to_abc Transformation
      settings: SourceProductBaseCode=PS
  freq : Constant  Value=50*2*pi
  vref : Outport  SampleTime=Ts
  Ome : Outport  Port=2  SampleTime=Ts
  wires:
  Pmeas/1 -> P controller/1(ERR)
  Qmeas/1 -> Q controller/1(E)
  Constant2/1 -> Mux6/2
  Constant1/1 -> Mux6/3
  Mux6/1 -> THREE PHASE REFERENCE GENERATOR/1
  Fcn/1 -> Mux3/1
  Fcn1/1 -> Mux3/2
  THREE PHASE REFERENCE GENERATOR/1 -> vref/1
  Mux3/1 -> THREE PHASE REFERENCE GENERATOR/2
  Q controller/1(Qout) -> Sum/1
  P controller/1(Pout) -> Sum1/1
  [EE] -> Sum/2
  Sum/1 -> Mux6/1
  freq/1 -> Sum1/2
  Sum1/1 -> Discrete-Time Integrator/1, Ome/1
  Discrete-Time Integrator/1 -> Fcn/1, Fcn1/1

== system Sim7/Control System2/Power Calculator ==
  ioal-bet : Inport
  Val_bet : Inport  Port=2
  Filter 1Hz 1MHz : Subsystem  Tag=FilterWizardSubSystem
      settings: ErrorFcn=dspFilterRealizedInBasicElemsAlgLoopErrFcnCallback
  Filter 1Hz 1MHz1 : Subsystem  Tag=FilterWizardSubSystem
      settings: ErrorFcn=dspFilterRealizedInBasicElemsAlgLoopErrFcnCallback
  Instantaneous active power1 : Fcn  Expr=u(1)*u(3)+u(2)*u(4)
  Instantaneous reactive power1 : Fcn  Expr=(-u(1)*u(4)+u(2)*u(3))
  Mux9 : Mux  Inputs=2
  Ppos : Outport
  Qpos : Outport  Port=2
  wires:
  Instantaneous active power1/1 -> Filter 1Hz 1MHz/1(Input)
  Mux9/1 -> Instantaneous active power1/1, Instantaneous reactive power1/1
  Instantaneous reactive power1/1 -> Filter 1Hz 1MHz1/1(Input)
  Val_bet/1 -> Mux9/1
  ioal-bet/1 -> Mux9/2
  Filter 1Hz 1MHz/1(Output) -> Ppos/1
  Filter 1Hz 1MHz1/1(Output) -> Qpos/1

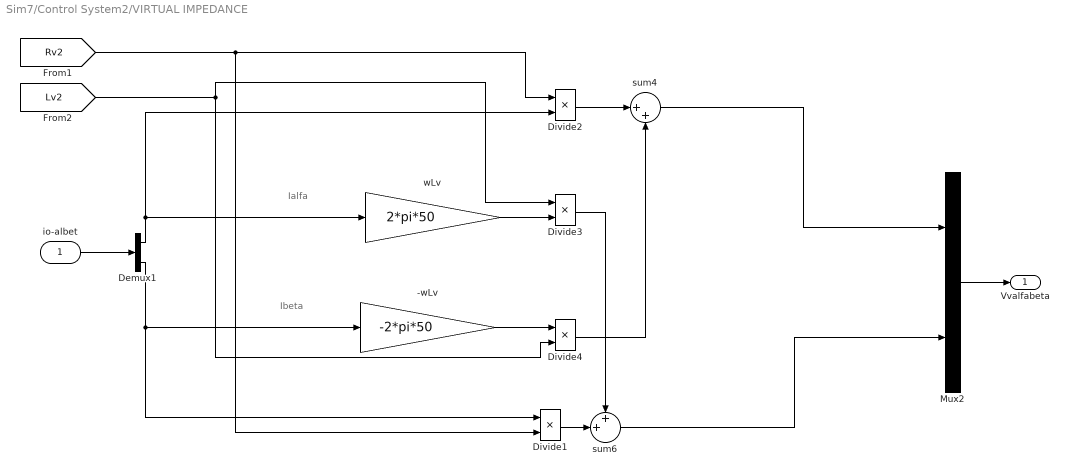
== system Sim7/Control System2/VIRTUAL IMPEDANCE ==
  note: Ialfa
  note: Ibeta
  io-albet : Inport
  -wLv : Gain  Gain=-2*pi*50
  Demux1 : Demux  Outputs=2
  Divide{1..4} (4 alike) : Product  Inputs=**  OutDataTypeStr=Inherit: Same as first input
  Mux2 : Mux  Inputs=2
  sum4 : Sum  Inputs=|++  InputSameDT=on  SaturateOnIntegerOverflow=on  OutDataTypeStr=Inherit: Same as first input
  sum6 : Sum  Inputs=++|  InputSameDT=on  SaturateOnIntegerOverflow=on  OutDataTypeStr=Inherit: Same as first input
  wLv : Gain  Gain=2*pi*50
  Vvalfabeta : Outport
  wires:
  Divide2/1 -> sum4/1
  Divide1/1 -> sum6/2
  wLv/1 -> Divide3/2
  Divide3/1 -> sum6/1
  [Lv2] -> Divide3/1, Divide4/2
  -wLv/1 -> Divide4/1
  Divide4/1 -> sum4/2
  Mux2/1 -> Vvalfabeta/1
  Demux1/2 -> -wLv/1, Divide1/1
  Demux1/1 -> wLv/1, Divide2/2
  [Rv2] -> Divide2/1, Divide1/2
  sum6/1 -> Mux2/2
  io-albet/1 -> Demux1/1
  sum4/1 -> Mux2/1

== system Sim7/Control System2/Voltage and Current Controller ==
  Valphabeta-error : Inport
  Iinv-alpha-beta : Inport  Port=2
  ome : Inport  Port=3
  Current Controller : Subsystem
  Sum3 : Sum  Inputs=|+-  SaturateOnIntegerOverflow=on
  Voltage Controller : Subsystem
  Ualphabeta_PR : Outport
  wires:
  Iinv-alpha-beta/1 -> Sum3/2
  ome/1 -> Current Controller/2(Ome), Voltage Controller/2(Ome)
  Valphabeta-error/1 -> Voltage Controller/1(Val_bet-error)
  Current Controller/1(Valbet-ref) -> Ualphabeta_PR/1
  Sum3/1 -> Current Controller/1(Ial_bet-error)
  Voltage Controller/1(Ialbet-ref) -> Sum3/1

== system Sim7/Control System/Droop Control/P controller ==
  ERR : Inport  SampleTime=Ts
  Divide2 : Product  Inputs=**  SampleTime=Ts  OutDataTypeStr=Inherit: Same as first input
  Pout : Outport
  wires:
  Divide2/1 -> Pout/1
  ERR/1 -> Divide2/2
  [KpP1] -> Divide2/1

== system Sim7/Control System/Droop Control/Q controller ==
  E : Inport  SampleTime=Ts
  Divide2 : Product  Inputs=**  OutDataTypeStr=Inherit: Same as first input
  Qout : Outport
  wires:
  E/1 -> Divide2/2
  [KpQ1] -> Divide2/1
  Divide2/1 -> Qout/1

== system Sim7/Control System/Power Calculator/Filter 1Hz 1MHz ==
  Input : Inport
  Delay11 : Delay  DelayLength=1  InitialCondition=0
  SumA21 : Sum  Inputs=|+-  RndMeth=Nearest  SaturateOnIntegerOverflow=on  OutDataTypeStr=Inherit: Same as first input
  SumB21 : Sum  Inputs=|++  RndMeth=Nearest  SaturateOnIntegerOverflow=on  OutDataTypeStr=Inherit: Same as first input
  a(2)(1) : Gain  Gain=-0.99999371683443194  ParamDataTypeStr=float('double')  RndMeth=Nearest  SaturateOnIntegerOverflow=on  OutDataTypeStr=Inherit: Same as input
  s(1) : Gain  Gain=3.1415827840267336e-006  ParamDataTypeStr=float('double')  RndMeth=Nearest  SaturateOnIntegerOverflow=on  OutDataTypeStr=Inherit: Same as input
  Output : Outport
  wires:
  Input/1 -> s(1)/1
  s(1)/1 -> SumA21/1
  SumA21/1 -> SumB21/1, Delay11/1
  SumB21/1 -> Output/1
  a(2)(1)/1 -> SumA21/2
  Delay11/1 -> a(2)(1)/1, SumB21/2

== system Sim7/Control System/Power Calculator/Filter 1Hz 1MHz1 ==
  Input : Inport
  Delay11 : Delay  DelayLength=1  InitialCondition=0
  SumA21 : Sum  Inputs=|+-  RndMeth=Nearest  SaturateOnIntegerOverflow=on  OutDataTypeStr=Inherit: Same as first input
  SumB21 : Sum  Inputs=|++  RndMeth=Nearest  SaturateOnIntegerOverflow=on  OutDataTypeStr=Inherit: Same as first input
  a(2)(1) : Gain  Gain=-0.99999371683443194  ParamDataTypeStr=float('double')  RndMeth=Nearest  SaturateOnIntegerOverflow=on  OutDataTypeStr=Inherit: Same as input
  s(1) : Gain  Gain=3.1415827840267336e-006  ParamDataTypeStr=float('double')  RndMeth=Nearest  SaturateOnIntegerOverflow=on  OutDataTypeStr=Inherit: Same as input
  Output : Outport
  wires:
  Delay11/1 -> SumB21/2, a(2)(1)/1
  a(2)(1)/1 -> SumA21/2
  SumB21/1 -> Output/1
  SumA21/1 -> Delay11/1, SumB21/1
  s(1)/1 -> SumA21/1
  Input/1 -> s(1)/1

== system Sim7/Control System/Voltage and Current Controller /Current Controller ==
  Ial_bet-error : Inport  SampleTime=Ts
  Ome : Inport  Port=2  SampleTime=Ts
  Demux2 : Demux  Outputs=2
  Mux2 : Mux  Inputs=2
  PR controller - alpha : Subsystem
  PR controller - beta : Subsystem
  Valbet-ref : Outport
  wires:
  Ial_bet-error/1 -> Demux2/1
  [KpI] -> PR controller - beta/2(KpI), PR controller - alpha/2(KpI)
  [KI1] -> PR controller - beta/3(KI1), PR controller - alpha/3(KI1)
  Ome/1 -> PR controller - beta/4(Ome), PR controller - alpha/4(Ome)
  [RSTT] -> PR controller - beta/5(Reset), PR controller - alpha/5(Reset)
  Demux2/1 -> PR controller - alpha/1(Ialpha_error)
  Mux2/1 -> Valbet-ref/1
  PR controller - alpha/1(Valpha-ref) -> Mux2/1
  PR controller - beta/1(Vbeta-ref) -> Mux2/2
  [wci1] -> PR controller - beta/6(wc1), PR controller - alpha/6(wc1)
  Demux2/2 -> PR controller - beta/1(Ibeta_error)

== system Sim7/Control System/Voltage and Current Controller /Voltage Controller ==
  Val_bet-error : Inport  SampleTime=Ts
  Ome : Inport  Port=2  SampleTime=Ts
  Demux2 : Demux  Outputs=2
  Mux2 : Mux  Inputs=2
  PR controller - alpha : Subsystem
  PR controller - beta : Subsystem
  Ialbet-ref : Outport
  wires:
  Val_bet-error/1 -> Demux2/1
  [KpV] -> PR controller - beta/2(KpV), PR controller - alpha/2(KpV)
  [KV1] -> PR controller - beta/3(KV1), PR controller - alpha/3(KV1)
  Ome/1 -> PR controller - beta/4(Ome), PR controller - alpha/4(Ome)
  [RSTT] -> PR controller - alpha/5(Reset), PR controller - beta/5(Reset)
  Demux2/1 -> PR controller - alpha/1(Valpha_error)
  Mux2/1 -> Ialbet-ref/1
  PR controller - alpha/1(Ialpha-ref) -> Mux2/1
  PR controller - beta/1(Ibeta-ref) -> Mux2/2
  [wcv1] -> PR controller - alpha/6(wc1), PR controller - beta/6(wc1)
  Demux2/2 -> PR controller - beta/1(Vbeta_error)

== system Sim7/Control System2/Droop Control/P controller ==
  ERR : Inport  SampleTime=Ts
  Divide2 : Product  Inputs=**  SampleTime=Ts  OutDataTypeStr=Inherit: Same as first input
  Pout : Outport
  wires:
  Divide2/1 -> Pout/1
  ERR/1 -> Divide2/2
  [KpP2] -> Divide2/1

== system Sim7/Control System2/Droop Control/Q controller ==
  E : Inport  SampleTime=Ts
  Divide2 : Product  Inputs=**  OutDataTypeStr=Inherit: Same as first input
  Qout : Outport
  wires:
  E/1 -> Divide2/2
  [KpQ2] -> Divide2/1
  Divide2/1 -> Qout/1

== system Sim7/Control System2/Power Calculator/Filter 1Hz 1MHz ==
  Input : Inport
  Delay11 : Delay  DelayLength=1  InitialCondition=0
  SumA21 : Sum  Inputs=|+-  RndMeth=Nearest  SaturateOnIntegerOverflow=on  OutDataTypeStr=Inherit: Same as first input
  SumB21 : Sum  Inputs=|++  RndMeth=Nearest  SaturateOnIntegerOverflow=on  OutDataTypeStr=Inherit: Same as first input
  a(2)(1) : Gain  Gain=-0.99999371683443194  ParamDataTypeStr=float('double')  RndMeth=Nearest  SaturateOnIntegerOverflow=on  OutDataTypeStr=Inherit: Same as input
  s(1) : Gain  Gain=3.1415827840267336e-006  ParamDataTypeStr=float('double')  RndMeth=Nearest  SaturateOnIntegerOverflow=on  OutDataTypeStr=Inherit: Same as input
  Output : Outport
  wires:
  Input/1 -> s(1)/1
  s(1)/1 -> SumA21/1
  SumA21/1 -> SumB21/1, Delay11/1
  SumB21/1 -> Output/1
  a(2)(1)/1 -> SumA21/2
  Delay11/1 -> a(2)(1)/1, SumB21/2

== system Sim7/Control System2/Power Calculator/Filter 1Hz 1MHz1 ==
  Input : Inport
  Delay11 : Delay  DelayLength=1  InitialCondition=0
  SumA21 : Sum  Inputs=|+-  RndMeth=Nearest  SaturateOnIntegerOverflow=on  OutDataTypeStr=Inherit: Same as first input
  SumB21 : Sum  Inputs=|++  RndMeth=Nearest  SaturateOnIntegerOverflow=on  OutDataTypeStr=Inherit: Same as first input
  a(2)(1) : Gain  Gain=-0.99999371683443194  ParamDataTypeStr=float('double')  RndMeth=Nearest  SaturateOnIntegerOverflow=on  OutDataTypeStr=Inherit: Same as input
  s(1) : Gain  Gain=3.1415827840267336e-006  ParamDataTypeStr=float('double')  RndMeth=Nearest  SaturateOnIntegerOverflow=on  OutDataTypeStr=Inherit: Same as input
  Output : Outport
  wires:
  Delay11/1 -> SumB21/2, a(2)(1)/1
  a(2)(1)/1 -> SumA21/2
  SumB21/1 -> Output/1
  SumA21/1 -> Delay11/1, SumB21/1
  s(1)/1 -> SumA21/1
  Input/1 -> s(1)/1

== system Sim7/Control System2/Voltage and Current Controller/Current Controller ==
  Ial_bet-error : Inport  SampleTime=Ts
  Ome : Inport  Port=2  SampleTime=Ts
  Demux2 : Demux  Outputs=2
  Mux2 : Mux  Inputs=2
  PR controller - alpha : Subsystem
  PR controller - beta : Subsystem
  Valbet-ref : Outport
  wires:
  Ial_bet-error/1 -> Demux2/1
  [KpI] -> PR controller - beta/2(KpI), PR controller - alpha/2(KpI)
  [KI1] -> PR controller - beta/3(KI1), PR controller - alpha/3(KI1)
  Ome/1 -> PR controller - beta/4(Ome), PR controller - alpha/4(Ome)
  [RSTT2] -> PR controller - beta/5(Reset), PR controller - alpha/5(Reset)
  Demux2/1 -> PR controller - alpha/1(Ialpha_error)
  Mux2/1 -> Valbet-ref/1
  PR controller - alpha/1(Valpha-ref) -> Mux2/1
  PR controller - beta/1(Vbeta-ref) -> Mux2/2
  [wci1] -> PR controller - beta/6(wc1), PR controller - alpha/6(wc1)
  Demux2/2 -> PR controller - beta/1(Ibeta_error)

== system Sim7/Control System2/Voltage and Current Controller/Voltage Controller ==
  Val_bet-error : Inport  SampleTime=Ts
  Ome : Inport  Port=2  SampleTime=Ts
  Demux2 : Demux  Outputs=2
  Mux2 : Mux  Inputs=2
  PR controller - alpha : Subsystem
  PR controller - beta : Subsystem
  Ialbet-ref : Outport
  wires:
  Val_bet-error/1 -> Demux2/1
  [KpV] -> PR controller - beta/2(KpV), PR controller - alpha/2(KpV)
  [KV1] -> PR controller - beta/3(KV1), PR controller - alpha/3(KV1)
  Ome/1 -> PR controller - beta/4(Ome), PR controller - alpha/4(Ome)
  [RSTT2] -> PR controller - alpha/5(Reset), PR controller - beta/5(Reset)
  Demux2/1 -> PR controller - alpha/1(Valpha_error)
  Mux2/1 -> Ialbet-ref/1
  PR controller - alpha/1(Ialpha-ref) -> Mux2/1
  PR controller - beta/1(Ibeta-ref) -> Mux2/2
  [wcv1] -> PR controller - alpha/6(wc1), PR controller - beta/6(wc1)
  Demux2/2 -> PR controller - beta/1(Vbeta_error)

== system Sim7/Control System/Voltage and Current Controller /Current Controller/PR controller - alpha ==
  Ialpha_error : Inport  SampleTime=Ts
  KpI : Inport  Port=2  SampleTime=Ts
  KI1 : Inport  Port=3  SampleTime=Ts
  Ome : Inport  Port=4  SampleTime=Ts
  Reset : Inport  Port=5  SampleTime=Ts
  wc1 : Inport  Port=6  SampleTime=Ts
  2*wc1 : Gain  Gain=2  SaturateOnIntegerOverflow=on  OutDataTypeStr=Inherit: Same as input  ParamDataTypeStr=Inherit: Same as input
  Divide1 : Product  Inputs=**  SampleTime=Ts  OutDataTypeStr=Inherit: Same as first input
  Divide2 : Product  Inputs=**  SampleTime=Ts  OutDataTypeStr=Inherit: Same as first input
  Math Function4 : Math  Operator=square  SignedPower=on  SampleTime=Ts  SaturateOnIntegerOverflow=on
  RES1 : Subsystem
  Sum3 : Sum  Inputs=2  SaturateOnIntegerOverflow=on
  Valpha-ref : Outport
  wires:
  Reset/1 -> RES1/2(RST)
  KI1/1 -> Divide2/1
  KpI/1 -> Divide1/1
  Ialpha_error/1 -> Divide1/2, Divide2/2
  Math Function4/1 -> RES1/3(om)
  Ome/1 -> Math Function4/1
  Sum3/1 -> Valpha-ref/1
  Divide2/1 -> RES1/1(In)
  Divide1/1 -> Sum3/1
  RES1/1(Out) -> Sum3/2
  wc1/1 -> 2*wc1/1
  2*wc1/1 -> RES1/4(om_C)

== system Sim7/Control System/Voltage and Current Controller /Current Controller/PR controller - beta ==
  Ibeta_error : Inport  SampleTime=Ts
  KpI : Inport  Port=2  SampleTime=Ts
  KI1 : Inport  Port=3  SampleTime=Ts
  Ome : Inport  Port=4  SampleTime=Ts
  Reset : Inport  Port=5  SampleTime=Ts
  wc1 : Inport  Port=6  SampleTime=Ts
  2*wc1 : Gain  Gain=2  SaturateOnIntegerOverflow=on  OutDataTypeStr=Inherit: Same as input  ParamDataTypeStr=Inherit: Same as input
  Divide1 : Product  Inputs=**  SampleTime=Ts  OutDataTypeStr=Inherit: Same as first input
  Divide2 : Product  Inputs=**  SampleTime=Ts  OutDataTypeStr=Inherit: Same as first input
  Math Function4 : Math  Operator=square  SignedPower=on  SampleTime=Ts  SaturateOnIntegerOverflow=on
  RES1 : Subsystem
  Sum3 : Sum  Inputs=2  SaturateOnIntegerOverflow=on
  Vbeta-ref : Outport
  wires:
  Reset/1 -> RES1/2(RST)
  KI1/1 -> Divide2/1
  KpI/1 -> Divide1/1
  Ibeta_error/1 -> Divide1/2, Divide2/2
  Math Function4/1 -> RES1/3(om)
  Ome/1 -> Math Function4/1
  Sum3/1 -> Vbeta-ref/1
  Divide2/1 -> RES1/1(In)
  Divide1/1 -> Sum3/1
  RES1/1(Out) -> Sum3/2
  wc1/1 -> 2*wc1/1
  2*wc1/1 -> RES1/4(om_C)

== system Sim7/Control System/Voltage and Current Controller /Voltage Controller/PR controller - alpha ==
  Valpha_error : Inport  SampleTime=Ts
  KpV : Inport  Port=2  SampleTime=Ts
  KV1 : Inport  Port=3  SampleTime=Ts
  Ome : Inport  Port=4  SampleTime=Ts
  Reset : Inport  Port=5  SampleTime=Ts
  wc1 : Inport  Port=6  SampleTime=Ts
  2*wc1 : Gain  Gain=2  SaturateOnIntegerOverflow=on  OutDataTypeStr=Inherit: Same as input  ParamDataTypeStr=Inherit: Same as input
  Divide1 : Product  Inputs=**  SampleTime=Ts  OutDataTypeStr=Inherit: Same as first input
  Divide2 : Product  Inputs=**  SampleTime=Ts  OutDataTypeStr=Inherit: Same as first input
  Math Function4 : Math  Operator=square  SignedPower=on  SampleTime=Ts  SaturateOnIntegerOverflow=on
  RES1 : Subsystem
  Sum3 : Sum  Inputs=2  SaturateOnIntegerOverflow=on
  Ialpha-ref : Outport
  wires:
  Reset/1 -> RES1/2(RST)
  KV1/1 -> Divide2/1
  KpV/1 -> Divide1/1
  Valpha_error/1 -> Divide1/2, Divide2/2
  Math Function4/1 -> RES1/3(om)
  Ome/1 -> Math Function4/1
  Sum3/1 -> Ialpha-ref/1
  Divide2/1 -> RES1/1(In)
  Divide1/1 -> Sum3/1
  RES1/1(Out) -> Sum3/2
  wc1/1 -> 2*wc1/1
  2*wc1/1 -> RES1/4(om_C)

== system Sim7/Control System/Voltage and Current Controller /Voltage Controller/PR controller - beta ==
  Vbeta_error : Inport  SampleTime=Ts
  KpV : Inport  Port=2  SampleTime=Ts
  KV1 : Inport  Port=3  SampleTime=Ts
  Ome : Inport  Port=4  SampleTime=Ts
  Reset : Inport  Port=5  SampleTime=Ts
  wc1 : Inport  Port=6  SampleTime=Ts
  2*wc1 : Gain  Gain=2  SaturateOnIntegerOverflow=on  OutDataTypeStr=Inherit: Same as input  ParamDataTypeStr=Inherit: Same as input
  Divide1 : Product  Inputs=**  SampleTime=Ts  OutDataTypeStr=Inherit: Same as first input
  Divide2 : Product  Inputs=**  SampleTime=Ts  OutDataTypeStr=Inherit: Same as first input
  Math Function4 : Math  Operator=square  SignedPower=on  SampleTime=Ts  SaturateOnIntegerOverflow=on
  RES1 : Subsystem
  Sum3 : Sum  Inputs=2  SaturateOnIntegerOverflow=on
  Ibeta-ref : Outport
  wires:
  Reset/1 -> RES1/2(RST)
  KV1/1 -> Divide2/1
  KpV/1 -> Divide1/1
  Vbeta_error/1 -> Divide1/2, Divide2/2
  Math Function4/1 -> RES1/3(om)
  Ome/1 -> Math Function4/1
  Sum3/1 -> Ibeta-ref/1
  Divide2/1 -> RES1/1(In)
  Divide1/1 -> Sum3/1
  RES1/1(Out) -> Sum3/2
  wc1/1 -> 2*wc1/1
  2*wc1/1 -> RES1/4(om_C)

== system Sim7/Control System2/Voltage and Current Controller/Current Controller/PR controller - alpha ==
  Ialpha_error : Inport  SampleTime=Ts
  KpI : Inport  Port=2  SampleTime=Ts
  KI1 : Inport  Port=3  SampleTime=Ts
  Ome : Inport  Port=4  SampleTime=Ts
  Reset : Inport  Port=5  SampleTime=Ts
  wc1 : Inport  Port=6  SampleTime=Ts
  2*wc1 : Gain  Gain=2  SaturateOnIntegerOverflow=on  OutDataTypeStr=Inherit: Same as input  ParamDataTypeStr=Inherit: Same as input
  Divide1 : Product  Inputs=**  SampleTime=Ts  OutDataTypeStr=Inherit: Same as first input
  Divide2 : Product  Inputs=**  SampleTime=Ts  OutDataTypeStr=Inherit: Same as first input
  Math Function4 : Math  Operator=square  SignedPower=on  SampleTime=Ts  SaturateOnIntegerOverflow=on
  RES1 : Subsystem
  Sum3 : Sum  Inputs=2  SaturateOnIntegerOverflow=on
  Valpha-ref : Outport
  wires:
  Reset/1 -> RES1/2(RST)
  KI1/1 -> Divide2/1
  KpI/1 -> Divide1/1
  Ialpha_error/1 -> Divide1/2, Divide2/2
  Math Function4/1 -> RES1/3(om)
  Ome/1 -> Math Function4/1
  Sum3/1 -> Valpha-ref/1
  Divide2/1 -> RES1/1(In)
  Divide1/1 -> Sum3/1
  RES1/1(Out) -> Sum3/2
  wc1/1 -> 2*wc1/1
  2*wc1/1 -> RES1/4(om_C)

== system Sim7/Control System2/Voltage and Current Controller/Current Controller/PR controller - beta ==
  Ibeta_error : Inport  SampleTime=Ts
  KpI : Inport  Port=2  SampleTime=Ts
  KI1 : Inport  Port=3  SampleTime=Ts
  Ome : Inport  Port=4  SampleTime=Ts
  Reset : Inport  Port=5  SampleTime=Ts
  wc1 : Inport  Port=6  SampleTime=Ts
  2*wc1 : Gain  Gain=2  SaturateOnIntegerOverflow=on  OutDataTypeStr=Inherit: Same as input  ParamDataTypeStr=Inherit: Same as input
  Divide1 : Product  Inputs=**  SampleTime=Ts  OutDataTypeStr=Inherit: Same as first input
  Divide2 : Product  Inputs=**  SampleTime=Ts  OutDataTypeStr=Inherit: Same as first input
  Math Function4 : Math  Operator=square  SignedPower=on  SampleTime=Ts  SaturateOnIntegerOverflow=on
  RES1 : Subsystem
  Sum3 : Sum  Inputs=2  SaturateOnIntegerOverflow=on
  Vbeta-ref : Outport
  wires:
  Reset/1 -> RES1/2(RST)
  KI1/1 -> Divide2/1
  KpI/1 -> Divide1/1
  Ibeta_error/1 -> Divide1/2, Divide2/2
  Math Function4/1 -> RES1/3(om)
  Ome/1 -> Math Function4/1
  Sum3/1 -> Vbeta-ref/1
  Divide2/1 -> RES1/1(In)
  Divide1/1 -> Sum3/1
  RES1/1(Out) -> Sum3/2
  wc1/1 -> 2*wc1/1
  2*wc1/1 -> RES1/4(om_C)

== system Sim7/Control System2/Voltage and Current Controller/Voltage Controller/PR controller - alpha ==
  Valpha_error : Inport  SampleTime=Ts
  KpV : Inport  Port=2  SampleTime=Ts
  KV1 : Inport  Port=3  SampleTime=Ts
  Ome : Inport  Port=4  SampleTime=Ts
  Reset : Inport  Port=5  SampleTime=Ts
  wc1 : Inport  Port=6  SampleTime=Ts
  2*wc1 : Gain  Gain=2  SaturateOnIntegerOverflow=on  OutDataTypeStr=Inherit: Same as input  ParamDataTypeStr=Inherit: Same as input
  Divide1 : Product  Inputs=**  SampleTime=Ts  OutDataTypeStr=Inherit: Same as first input
  Divide2 : Product  Inputs=**  SampleTime=Ts  OutDataTypeStr=Inherit: Same as first input
  Math Function4 : Math  Operator=square  SignedPower=on  SampleTime=Ts  SaturateOnIntegerOverflow=on
  RES1 : Subsystem
  Sum3 : Sum  Inputs=2  SaturateOnIntegerOverflow=on
  Ialpha-ref : Outport
  wires:
  Reset/1 -> RES1/2(RST)
  KV1/1 -> Divide2/1
  KpV/1 -> Divide1/1
  Valpha_error/1 -> Divide1/2, Divide2/2
  Math Function4/1 -> RES1/3(om)
  Ome/1 -> Math Function4/1
  Sum3/1 -> Ialpha-ref/1
  Divide2/1 -> RES1/1(In)
  Divide1/1 -> Sum3/1
  RES1/1(Out) -> Sum3/2
  wc1/1 -> 2*wc1/1
  2*wc1/1 -> RES1/4(om_C)

== system Sim7/Control System2/Voltage and Current Controller/Voltage Controller/PR controller - beta ==
  Vbeta_error : Inport  SampleTime=Ts
  KpV : Inport  Port=2  SampleTime=Ts
  KV1 : Inport  Port=3  SampleTime=Ts
  Ome : Inport  Port=4  SampleTime=Ts
  Reset : Inport  Port=5  SampleTime=Ts
  wc1 : Inport  Port=6  SampleTime=Ts
  2*wc1 : Gain  Gain=2  SaturateOnIntegerOverflow=on  OutDataTypeStr=Inherit: Same as input  ParamDataTypeStr=Inherit: Same as input
  Divide1 : Product  Inputs=**  SampleTime=Ts  OutDataTypeStr=Inherit: Same as first input
  Divide2 : Product  Inputs=**  SampleTime=Ts  OutDataTypeStr=Inherit: Same as first input
  Math Function4 : Math  Operator=square  SignedPower=on  SampleTime=Ts  SaturateOnIntegerOverflow=on
  RES1 : Subsystem
  Sum3 : Sum  Inputs=2  SaturateOnIntegerOverflow=on
  Ibeta-ref : Outport
  wires:
  Reset/1 -> RES1/2(RST)
  KV1/1 -> Divide2/1
  KpV/1 -> Divide1/1
  Vbeta_error/1 -> Divide1/2, Divide2/2
  Math Function4/1 -> RES1/3(om)
  Ome/1 -> Math Function4/1
  Sum3/1 -> Ibeta-ref/1
  Divide2/1 -> RES1/1(In)
  Divide1/1 -> Sum3/1
  RES1/1(Out) -> Sum3/2
  wc1/1 -> 2*wc1/1
  2*wc1/1 -> RES1/4(om_C)
